simulink model "PC_MSFS_STATION"  (R2021b)
settings: Solver=FixedStepAuto  StartTime=0.0  StopTime=2000  FixedStep=0.03  RelTol=1e-3
undefined symbols (not defined in the file): CONTROL, DiscIntNeverNeededParam, f, MODEL, MODEL_INI
libraries: instrumentlib x42, SimConnectToolbox x6, simulink x4
(part 1 of 3)
settings Model: Creator=Andreas  LastModifiedBy=ae-dagbeyibor3
settings SolverCC: AlgebraicLoopSolver=TrustRegion
settings DebuggingCC: InheritedTsInSrcMsg=none  SFMachineParentedDataDiag=warning

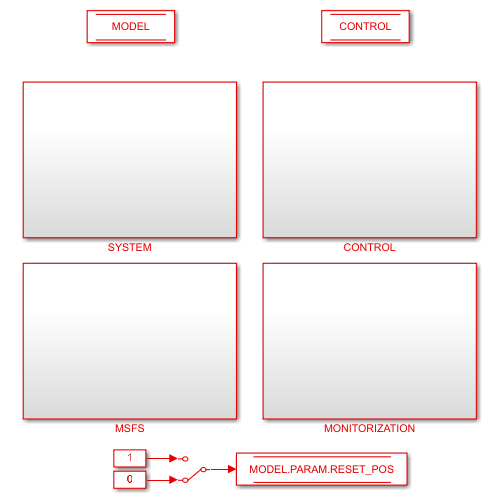
[thumbnail: Simulink's stored preview of the top-level diagram]
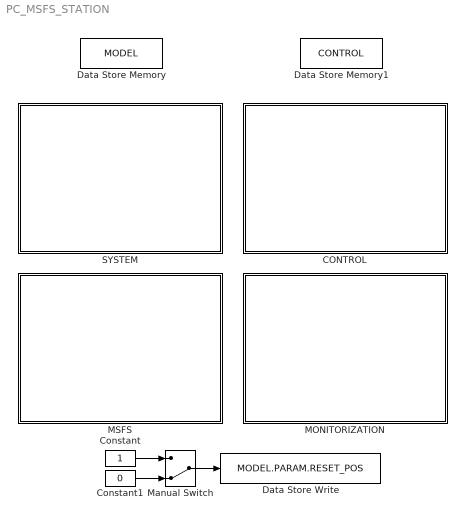
== system PC_MSFS_STATION ==
  CONTROL : Subsystem
  Constant : Constant  SampleTime=-1
  Constant1 : Constant  Value=0  SampleTime=-1
  Data Store Memory : DataStoreMemory  DataStoreName=MODEL  ReadBeforeWriteMsg=warning  WriteAfterWriteMsg=warning  WriteAfterReadMsg=warning  InitialValue=MODEL_INI  ShowAdditionalParam=off  OutDataTypeStr=Bus: MODEL_Bus
  Data Store Memory1 : DataStoreMemory  DataStoreName=CONTROL  ReadBeforeWriteMsg=warning  WriteAfterWriteMsg=warning  WriteAfterReadMsg=warning  InitialValue=CONTROL_INI  ShowAdditionalParam=off  OutDataTypeStr=Bus: CONTROL_Bus
  Data Store Write : DataStoreWrite  DataStoreName=MODEL  DataStoreElements=MODEL.PARAM.RESET_POS  IndexOptions=Index vector (dialog)  Indices=1  OutputSizes=1
  MONITORIZATION : Subsystem
  MSFS : Subsystem
  Manual Switch : ManualSwitch  CurrentSetting=0
  SYSTEM : Subsystem
  wires:
  Constant/1 -> Manual Switch/1
  Constant1/1 -> Manual Switch/2
  Manual Switch/1 -> Data Store Write/1

== system PC_MSFS_STATION/CONTROL ==
  ISR : Subsystem
  MEDEVAC : Subsystem  Commented=on

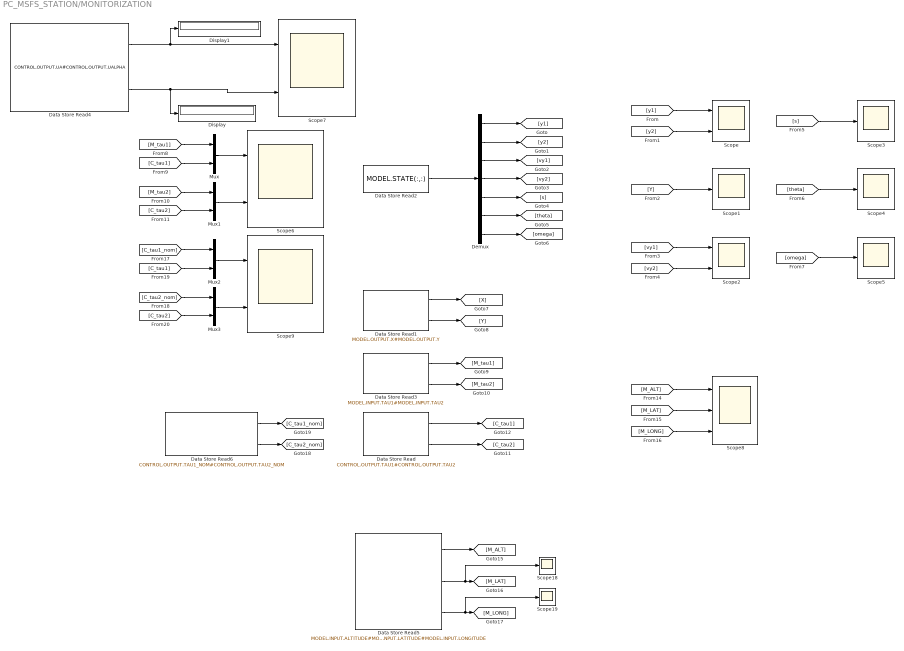
== system PC_MSFS_STATION/MONITORIZATION ==
  Data Store Read : DataStoreRead  DataStoreName=CONTROL  DataStoreElements=CONTROL.OUTPUT.TAU1#CONTROL.OUTPUT.TAU2  IndexOptions=Index vector (dialog)  Indices=1  OutputSizes=1
  Data Store Read1 : DataStoreRead  DataStoreName=MODEL  SampleTime=MODEL_INI.PARAM.SIM_SAMPLING_TIME  DataStoreElements=MODEL.OUTPUT.X#MODEL.OUTPUT.Y  IndexOptions=Index vector (dialog)  Indices=1  OutputSizes=1
  Data Store Read2 : DataStoreRead  DataStoreName=MODEL  SampleTime=MODEL_INI.PARAM.SIM_SAMPLING_TIME  DataStoreElements=MODEL.STATE(:,:)  IndexOptions=Index vector (dialog)  Indices=1  OutputSizes=1
  Data Store Read3 : DataStoreRead  DataStoreName=MODEL  SampleTime=MODEL_INI.PARAM.SIM_SAMPLING_TIME  DataStoreElements=MODEL.INPUT.TAU1#MODEL.INPUT.TAU2  IndexOptions=Index vector (dialog)  Indices=1  OutputSizes=1
  Data Store Read4 : DataStoreRead  DataStoreName=CONTROL  DataStoreElements=CONTROL.OUTPUT.UA#CONTROL.OUTPUT.UALPHA  IndexOptions=Index vector (dialog)  Indices=1  OutputSizes=1
  Data Store Read5 : DataStoreRead  DataStoreName=MODEL  SampleTime=MODEL_INI.PARAM.SIM_SAMPLING_TIME  DataStoreElements=MODEL.INPUT.ALTITUDE#MODEL.INPUT.LATITUDE#MODEL.INPUT.LONGITUDE  IndexOptions=Index vector (dialog)  Indices=1  OutputSizes=1
  Data Store Read6 : DataStoreRead  DataStoreName=CONTROL  DataStoreElements=CONTROL.OUTPUT.TAU1_NOM#CONTROL.OUTPUT.TAU2_NOM  IndexOptions=Index vector (dialog)  Indices=1  OutputSizes=1
  Demux : Demux  Outputs=7
  Display : Display
  Display1 : Display
  Mux{,1..3} (4 alike) : Mux  Inputs=2
  Scope{,2,6..7,9} (5 alike) : Scope  NumInputPorts=2
  Scope{1,3..5,18..19} (6 alike) : Scope
  Scope8 : Scope  NumInputPorts=3
  wires:
  Data Store Read2/1 -> Demux/1
  Demux/1 -> [y1]
  Demux/2 -> [y2]
  Demux/3 -> [vy1]
  Demux/4 -> [vy2]
  Demux/5 -> [s]
  Demux/6 -> [theta]
  Demux/7 -> [omega]
  [y1] -> Scope/1
  [y2] -> Scope/2
  Data Store Read1/1 -> [X]
  Data Store Read1/2 -> [Y]
  [Y] -> Scope1/1
  [vy2] -> Scope2/2
  [vy1] -> Scope2/1
  [s] -> Scope3/1
  [theta] -> Scope4/1
  [omega] -> Scope5/1
  Data Store Read3/1 -> [M_tau1]
  Data Store Read3/2 -> [M_tau2]
  Data Store Read/1 -> [C_tau1]
  Data Store Read/2 -> [C_tau2]
  Mux/1 -> Scope6/1
  Mux1/1 -> Scope6/2
  [M_tau1] -> Mux/1
  [M_tau2] -> Mux1/1
  [C_tau2] -> Mux1/2
  [C_tau1] -> Mux/2
  Data Store Read5/2 -> Scope18/1, [M_LAT]
  Data Store Read5/1 -> [M_ALT]
  Data Store Read5/3 -> Scope19/1, [M_LONG]
  [M_LAT] -> Scope8/2
  [M_ALT] -> Scope8/1
  [M_LONG] -> Scope8/3
  Data Store Read6/2 -> [C_tau2_nom]
  Data Store Read6/1 -> [C_tau1_nom]
  [C_tau1] -> Mux2/2
  [C_tau2] -> Mux3/2
  [C_tau2_nom] -> Mux3/1
  [C_tau1_nom] -> Mux2/1
  Mux3/1 -> Scope9/2
  Mux2/1 -> Scope9/1
  Data Store Read4/1 -> Display1/1, Scope7/1
  Data Store Read4/2 -> Display/1, Scope7/2

== system PC_MSFS_STATION/MSFS ==
  ISR : Subsystem
  MEDEVAC : Subsystem  Commented=on

== system PC_MSFS_STATION/SYSTEM ==
  ISR : Subsystem
  MEDEVAC : Subsystem  Commented=on

== system PC_MSFS_STATION/CONTROL/ISR ==
  Bus Selector : BusSelector  OutputSignals=STATE,INPUT.ALTITUDE
  Bus Selector1 : BusSelector  OutputSignals=PARAM.ALTITUDE
  CONTROL UPDATE : MATLAB Function  TreatAsAtomicUnit=on
  Data Store Read : DataStoreRead  DataStoreName=CONTROL  SampleTime=MODEL_INI.PARAM.SIM_SAMPLING_TIME  IndexOptions=Index vector (dialog)  Indices=1  OutputSizes=1
  Data Store Read1 : DataStoreRead  DataStoreName=MODEL  SampleTime=MODEL_INI.PARAM.SIM_SAMPLING_TIME  IndexOptions=Index vector (dialog)  Indices=1  OutputSizes=1
  Data Store Write : DataStoreWrite  DataStoreName=CONTROL  IndexOptions=Index vector (dialog)  Indices=1  OutputSizes=1
  Display : Display
  Scope : Scope
  Scope1 : Scope
  wires:
  Data Store Read1/1 -> Bus Selector/1
  Bus Selector1/1 -> Display/1, Scope1/1  "<ALTITUDE>"
  Data Store Read/1 -> CONTROL UPDATE/1(CONTROL_IN)
  CONTROL UPDATE/1(CONTROL) -> Bus Selector1/1, Data Store Write/1
  Bus Selector/1 -> CONTROL UPDATE/2(STATE)  "<STATE>"
  Bus Selector/2 -> CONTROL UPDATE/3(ALTITUDE_IN), Scope/1  "<ALTITUDE>"

== system PC_MSFS_STATION/CONTROL/MEDEVAC ==
  Bus Selector : BusSelector  OutputSignals=STATE,INPUT.ALTITUDE
  Bus Selector1 : BusSelector  OutputSignals=PARAM.ALTITUDE
  CONTROL UPDATE : MATLAB Function  TreatAsAtomicUnit=on
  Data Store Read : DataStoreRead  DataStoreName=CONTROL  SampleTime=MODEL_INI.PARAM.SIM_SAMPLING_TIME  IndexOptions=Index vector (dialog)  Indices=1  OutputSizes=1
  Data Store Read1 : DataStoreRead  DataStoreName=MODEL  SampleTime=MODEL_INI.PARAM.SIM_SAMPLING_TIME  IndexOptions=Index vector (dialog)  Indices=1  OutputSizes=1
  Data Store Write : DataStoreWrite  DataStoreName=CONTROL  IndexOptions=Index vector (dialog)  Indices=1  OutputSizes=1
  Display : Display
  Scope : Scope
  Scope1 : Scope
  wires:
  Bus Selector/2 -> Scope/1, CONTROL UPDATE/3(ALTITUDE_IN)  "<ALTITUDE>"
  Bus Selector/1 -> CONTROL UPDATE/2(STATE)  "<STATE>"
  CONTROL UPDATE/1(CONTROL) -> Data Store Write/1, Bus Selector1/1
  Data Store Read/1 -> CONTROL UPDATE/1(CONTROL_IN)
  Bus Selector1/1 -> Scope1/1, Display/1  "<ALTITUDE>"
  Data Store Read1/1 -> Bus Selector/1

== system PC_MSFS_STATION/MSFS/ISR ==
  COMMUNICATIONS : Subsystem
  Compare To Constant1 : simulink/Logic and Bit Operations/Compare To Constant  relop=>  const=0  OutDataTypeStr=boolean
  Compare To Constant4 : simulink/Logic and Bit Operations/Compare To Constant  relop===  const=0  OutDataTypeStr=boolean
  Data Store Read1 : DataStoreRead  DataStoreName=CONTROL  DataStoreElements=CONTROL.PARAM.FLIGHT_STATUS  IndexOptions=Index vector (dialog)  Indices=1  OutputSizes=1
  Data Store Read4 : DataStoreRead  DataStoreName=CONTROL  DataStoreElements=CONTROL.PARAM.FLIGHT_STATUS  IndexOptions=Index vector (dialog)  Indices=1  OutputSizes=1
  IN FLIGHT : Subsystem
  TAKE OFF TRIM : Subsystem
  wires:
  Data Store Read4/1 -> Compare To Constant4/1
  Compare To Constant1/1 -> IN FLIGHT/Enable
  Compare To Constant4/1 -> TAKE OFF TRIM/Enable
  Data Store Read1/1 -> Compare To Constant1/1

== system PC_MSFS_STATION/MSFS/MEDEVAC ==
  COMMUNICATIONS : Subsystem
  Compare To Constant1 : simulink/Logic and Bit Operations/Compare To Constant  relop=>  const=0  OutDataTypeStr=boolean
  Compare To Constant4 : simulink/Logic and Bit Operations/Compare To Constant  relop===  const=0  OutDataTypeStr=boolean
  Data Store Read1 : DataStoreRead  DataStoreName=CONTROL  DataStoreElements=CONTROL.PARAM.FLIGHT_STATUS  IndexOptions=Index vector (dialog)  Indices=1  OutputSizes=1
  Data Store Read4 : DataStoreRead  DataStoreName=CONTROL  DataStoreElements=CONTROL.PARAM.FLIGHT_STATUS  IndexOptions=Index vector (dialog)  Indices=1  OutputSizes=1
  IN FLIGHT : Subsystem
  TAKE OFF TRIM : Subsystem
  wires:
  Data Store Read1/1 -> Compare To Constant1/1
  Compare To Constant4/1 -> TAKE OFF TRIM/Enable
  Compare To Constant1/1 -> IN FLIGHT/Enable
  Data Store Read4/1 -> Compare To Constant4/1

== system PC_MSFS_STATION/SYSTEM/ISR ==
  Bus Selector2 : BusSelector  OutputSignals=OUTPUT.TAU1,OUTPUT.TAU2
  Bus Selector3 : BusSelector  OutputSignals=PARAM.FLIGHT_STATUS
  Data Store Read2 : DataStoreRead  DataStoreName=MODEL  SampleTime=MODEL_INI.PARAM.SIM_SAMPLING_TIME  IndexOptions=Index vector (dialog)  Indices=1  OutputSizes=1
  Data Store Read3 : DataStoreRead  DataStoreName=CONTROL  IndexOptions=Index vector (dialog)  Indices=1  OutputSizes=1
  Data Store Read4 : DataStoreRead  DataStoreName=CONTROL  DataStoreElements=CONTROL.PARAM.ALTITUDE  IndexOptions=Index vector (dialog)  Indices=1  OutputSizes=1
  Data Store Read5 : DataStoreRead  DataStoreName=CONTROL  IndexOptions=Index vector (dialog)  Indices=1  OutputSizes=1
  Data Store Read6 : DataStoreRead  DataStoreName=MODEL  DataStoreElements=MODEL.PARAM.RESET_POS  IndexOptions=Index vector (dialog)  Indices=1  OutputSizes=1
  Data Store Read8 : DataStoreRead  DataStoreName=MODEL  DataStoreElements=MODEL.PARAM.INIT_STATE(:,:)  IndexOptions=Index vector (dialog)  Indices=1  OutputSizes=1
  Data Store Write : DataStoreWrite  DataStoreName=MODEL  IndexOptions=Index vector (dialog)  Indices=1  OutputSizes=1
  Data Store Write2 : DataStoreWrite  DataStoreName=MODEL  DataStoreElements=MODEL.INPUT.TAU1#MODEL.INPUT.TAU2  IndexOptions=Index vector (dialog)  Indices=1  OutputSizes=1
  Data Store Write3 : DataStoreWrite  DataStoreName=MODEL  DataStoreElements=MODEL.PARAM.FLIGHT_STATUS  IndexOptions=Index vector (dialog)  Indices=1  OutputSizes=1
  Data Store Write4 : DataStoreWrite  DataStoreName=MODEL  DataStoreElements=MODEL.OUTPUT.ALTITUDE  IndexOptions=Index vector (dialog)  Indices=1  OutputSizes=1
  Demux : Demux  Outputs=7
  Discrete-Time Integrator : DiscreteIntegrator  ExternalReset=rising  InitialConditionSource=external  SampleTime=-1  ICPrevOutput=DiscIntNeverNeededParam  ICPrevScaledInput=DiscIntNeverNeededParam
  Display{,1,10..11,16..20} (9 alike) : Display
  Scope{,1..5,10..14} (11 alike) : Scope
  UNICYCLE MODEL : MATLAB Function  TreatAsAtomicUnit=on
  wires:
  Discrete-Time Integrator/1 -> Demux/1, UNICYCLE MODEL/1(STATE)
  UNICYCLE MODEL/2(MODEL) -> Data Store Write/1
  Data Store Read8/1 -> Discrete-Time Integrator/3
  UNICYCLE MODEL/1(STATE_DERIVATIVE) -> Discrete-Time Integrator/1
  Bus Selector2/2 -> Scope2/1, Data Store Write2/2  "<TAU2>"
  Demux/3 -> Scope10/1, Display16/1
  Bus Selector3/1 -> Display1/1, Data Store Write3/1, Scope1/1  "<FLIGHT_STATUS>"
  Bus Selector2/1 -> Scope3/1, Data Store Write2/1  "<TAU1>"
  Data Store Read4/1 -> Display/1, Scope/1, Data Store Write4/1
  Data Store Read3/1 -> Bus Selector3/1
  Demux/6 -> Scope13/1, Display19/1
  Demux/5 -> Scope12/1, Display18/1
  Data Store Read5/1 -> Bus Selector2/1
  Demux/1 -> Scope4/1, Display10/1
  Demux/7 -> Scope14/1, Display20/1
  Demux/2 -> Scope5/1, Display11/1
  Data Store Read2/1 -> UNICYCLE MODEL/2(MODEL_IN)
  Demux/4 -> Scope11/1, Display17/1
  Data Store Read6/1 -> Discrete-Time Integrator/2

== system PC_MSFS_STATION/SYSTEM/MEDEVAC ==
  Bus Selector2 : BusSelector  OutputSignals=OUTPUT.TAU1,OUTPUT.TAU2
  Bus Selector3 : BusSelector  OutputSignals=PARAM.FLIGHT_STATUS
  Data Store Read2 : DataStoreRead  DataStoreName=MODEL  SampleTime=MODEL_INI.PARAM.SIM_SAMPLING_TIME  IndexOptions=Index vector (dialog)  Indices=1  OutputSizes=1
  Data Store Read3 : DataStoreRead  DataStoreName=CONTROL  IndexOptions=Index vector (dialog)  Indices=1  OutputSizes=1
  Data Store Read4 : DataStoreRead  DataStoreName=CONTROL  DataStoreElements=CONTROL.PARAM.ALTITUDE  IndexOptions=Index vector (dialog)  Indices=1  OutputSizes=1
  Data Store Read5 : DataStoreRead  DataStoreName=CONTROL  IndexOptions=Index vector (dialog)  Indices=1  OutputSizes=1
  Data Store Read6 : DataStoreRead  DataStoreName=MODEL  DataStoreElements=MODEL.PARAM.RESET_POS  IndexOptions=Index vector (dialog)  Indices=1  OutputSizes=1
  Data Store Read8 : DataStoreRead  DataStoreName=MODEL  DataStoreElements=MODEL.PARAM.INIT_STATE(:,:)  IndexOptions=Index vector (dialog)  Indices=1  OutputSizes=1
  Data Store Write : DataStoreWrite  DataStoreName=MODEL  IndexOptions=Index vector (dialog)  Indices=1  OutputSizes=1
  Data Store Write2 : DataStoreWrite  DataStoreName=MODEL  DataStoreElements=MODEL.INPUT.TAU1#MODEL.INPUT.TAU2  IndexOptions=Index vector (dialog)  Indices=1  OutputSizes=1
  Data Store Write3 : DataStoreWrite  DataStoreName=MODEL  DataStoreElements=MODEL.PARAM.FLIGHT_STATUS  IndexOptions=Index vector (dialog)  Indices=1  OutputSizes=1
  Data Store Write4 : DataStoreWrite  DataStoreName=MODEL  DataStoreElements=MODEL.OUTPUT.ALTITUDE  IndexOptions=Index vector (dialog)  Indices=1  OutputSizes=1
  Demux : Demux  Outputs=7
  Discrete-Time Integrator : DiscreteIntegrator  ExternalReset=rising  InitialConditionSource=external  SampleTime=-1  ICPrevOutput=DiscIntNeverNeededParam  ICPrevScaledInput=DiscIntNeverNeededParam
  Display{,1,10..11,16..20} (9 alike) : Display
  Scope{,1..5,10..14} (11 alike) : Scope
  UNICYCLE MODEL : MATLAB Function  TreatAsAtomicUnit=on
  wires:
  Data Store Read6/1 -> Discrete-Time Integrator/2
  Demux/4 -> Display17/1, Scope11/1
  Data Store Read2/1 -> UNICYCLE MODEL/2(MODEL_IN)
  Demux/2 -> Display11/1, Scope5/1
  Demux/7 -> Display20/1, Scope14/1
  Demux/1 -> Display10/1, Scope4/1
  Data Store Read5/1 -> Bus Selector2/1
  Demux/5 -> Display18/1, Scope12/1
  Demux/6 -> Display19/1, Scope13/1
  Data Store Read3/1 -> Bus Selector3/1
  Data Store Read4/1 -> Data Store Write4/1, Scope/1, Display/1
  Bus Selector2/1 -> Data Store Write2/1, Scope3/1  "<TAU1>"
  Bus Selector3/1 -> Scope1/1, Data Store Write3/1, Display1/1  "<FLIGHT_STATUS>"
  Demux/3 -> Display16/1, Scope10/1
  Bus Selector2/2 -> Data Store Write2/2, Scope2/1  "<TAU2>"
  UNICYCLE MODEL/1(STATE_DERIVATIVE) -> Discrete-Time Integrator/1
  Data Store Read8/1 -> Discrete-Time Integrator/3
  UNICYCLE MODEL/2(MODEL) -> Data Store Write/1
  Discrete-Time Integrator/1 -> UNICYCLE MODEL/1(STATE), Demux/1

== system PC_MSFS_STATION/MSFS/ISR/COMMUNICATIONS ==
  LOCAL COMMUNICATIONS : Subsystem  Commented=on
  SERVER COMMUNICATIONS : Subsystem

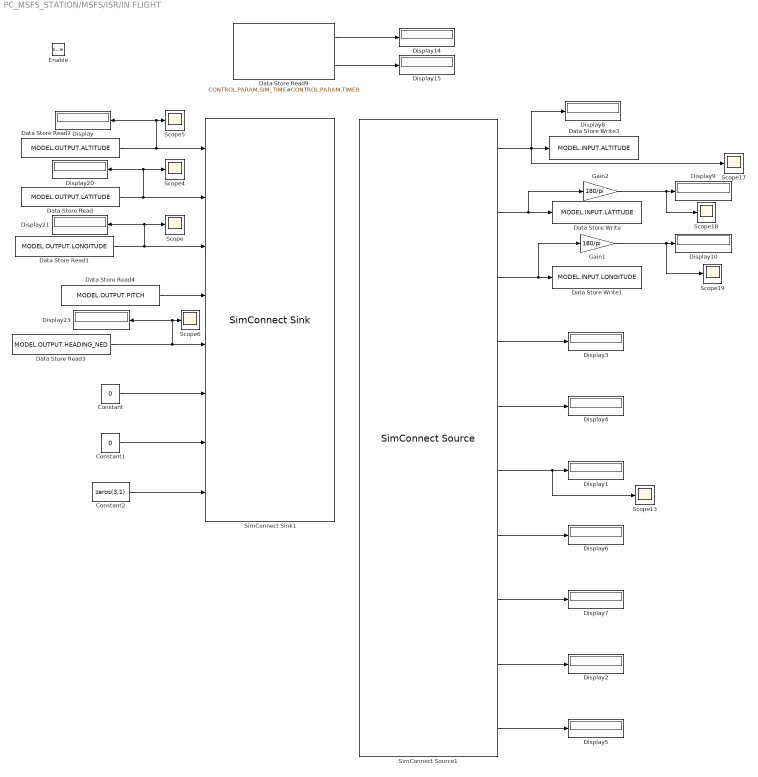
== system PC_MSFS_STATION/MSFS/ISR/IN FLIGHT ==
  Enable : EnablePort
  Constant : Constant  Value=0  SampleTime=-1
  Constant1 : Constant  Value=0  SampleTime=-1
  Constant2 : Constant  Value=zeros(3,1)  SampleTime=-1
  Data Store Read : DataStoreRead  DataStoreName=MODEL  DataStoreElements=MODEL.OUTPUT.LATITUDE  IndexOptions=Index vector (dialog)  Indices=1  OutputSizes=1
  Data Store Read1 : DataStoreRead  DataStoreName=MODEL  DataStoreElements=MODEL.OUTPUT.LONGITUDE  IndexOptions=Index vector (dialog)  Indices=1  OutputSizes=1
  Data Store Read2 : DataStoreRead  DataStoreName=MODEL  DataStoreElements=MODEL.OUTPUT.ALTITUDE  IndexOptions=Index vector (dialog)  Indices=1  OutputSizes=1
  Data Store Read3 : DataStoreRead  DataStoreName=MODEL  DataStoreElements=MODEL.OUTPUT.HEADING_NED  IndexOptions=Index vector (dialog)  Indices=1  OutputSizes=1
  Data Store Read4 : DataStoreRead  DataStoreName=MODEL  DataStoreElements=MODEL.OUTPUT.PITCH  IndexOptions=Index vector (dialog)  Indices=1  OutputSizes=1
  Data Store Read9 : DataStoreRead  DataStoreName=CONTROL  DataStoreElements=CONTROL.PARAM.SIM_TIME#CONTROL.PARAM.TIMER  IndexOptions=Index vector (dialog)  Indices=1  OutputSizes=1
  Data Store Write : DataStoreWrite  DataStoreName=MODEL  DataStoreElements=MODEL.INPUT.LATITUDE  IndexOptions=Index vector (dialog)  Indices=1  OutputSizes=1
  Data Store Write1 : DataStoreWrite  DataStoreName=MODEL  DataStoreElements=MODEL.INPUT.LONGITUDE  IndexOptions=Index vector (dialog)  Indices=1  OutputSizes=1
  Data Store Write3 : DataStoreWrite  DataStoreName=MODEL  DataStoreElements=MODEL.INPUT.ALTITUDE  IndexOptions=Index vector (dialog)  Indices=1  OutputSizes=1
  Display{,1..10,14..15,20..21,23} (16 alike) : Display
  Gain1 : Gain  Gain=180/pi
  Gain2 : Gain  Gain=180/pi
  Scope{,4..6,13,17..19} (8 alike) : Scope
  SimConnect Sink1 : SimConnectToolbox/SimConnect Sink  configurationIndex=0  connectionName=SimConnectSink  variables=|
      | PLANE ALTITUDE, FEET;
      | PLANE LATITUDE, RADIANS;
      | PLANE LONGITUDE, RADIANS;
      | PLANE PITCH DEGREES, RADIANS;
      | PLANE HEADING DEGREES TRUE, RADIANS;
      | PLANE BANK DEGREES, RADIANS;
      | AILERON POSITION, POSITION;
      | AILERON TRIM PCT, PERCENT;
      settings: SourceProductName=SimConnect Toolbox
      mask Display:
      | % This is a new mask on top of the base mask.
      | % Use "View base mask" link below to see the base mask.
      | %port_label('input', 1, 'Rudder Trim', 'texmode', 'on')
      | port_label('input', 1, 'PLANE ALTITUDE, FEET', 'texmode', 'on')
      | port_label('input', 2, 'PLANE LATITUDE, RADIANS', 'texmode', 'on')
      | port_label('input', 3, 'PLANE LONGITUDE, RADIANS', 'texmode', 'on')
      | port_label('input', 4, 'PITCH DEGREES, RADIANS', 'texmode', 'on')
      | port_label('input', 5, 'HEADING DEGREES TRUE, RADIANS', 'texmode', 'on')
      | port_label('input', 6, 'PLANE BANK DEGREES, RADIANS;', 'texmode', 'on')
      | port_label('input', 7, 'AILERON POSITION, POSITION', 'texmode', 'on')
      | port_label('input', 8, 'AILERON TRIM PCT, PERCENT OVER 100', 'texmode', 'on')
  SimConnect Source1 : SimConnectToolbox/SimConnect Source  configurationIndex=0  connectionName=SimConnectSource  variables=|
      | PLANE ALTITUDE, FEET;
      | PLANE LATITUDE, RADIANS;
      | PLANE LONGITUDE, RADIANS;
      | ROTATION VELOCITY BODY X, FEET PER SECOND;
      | PLANE PITCH DEGREES, RADIANS;
      | PLANE HEADING DEGREES TRUE, RADIANS;
      | PLANE HEADING DEGREES MAGNETIC, RADIANS;
      | PLANE HEADING DEGREES GYRO, DEGREES;
      | AILERON POSITION, POSITION;
      | AILERON TRIM PCT, PERCENT OVER 100;
      settings: SourceProductName=SimConnect Toolbox
      mask Display:
      | % This is a new mask on top of the base mask.
      | % Use "View base mask" link below to see the base mask.
      | % port_label('output', 1, 'g', 'texmode', 'on')
      | port_label('output', 1, 'PLANE ALTITUDE, FEET', 'texmode', 'on')
      | port_label('output', 2, 'PLANE LATITUDE, RADIANS', 'texmode', 'on')
      | port_label('output', 3, 'PLANE LONGITUDE, RADIANS', 'texmode', 'on')
      | port_label('output', 4, 'VELOCITY BODY X, FEET PER SECOND', 'texmode', 'on')
      | port_label('output', 5, 'PITCH DEGREES, RADIANS', 'texmode', 'on')
      | port_label('output', 6, 'HEADING DEGREES TRUE, RADIANS', 'texmode', 'on')
      | port_label('output', 7, 'HEADING DEGREES MAGNETIC, RADIANS', 'texmode', 'on')
      | port_label('output', 8, 'HEADING DEGREES GYRO, DEGREES', 'texmode', 'on')
      | port_label('output', 9, 'AILERON POSITION, POSITION', 'texmode', 'on')
      | port_label('output', 10, 'AILERON TRIM PCT, PERCENT OVER 100', 'texmode', 'on')
  wires:
  Constant2/1 -> SimConnect Sink1/8
  SimConnect Source1/9 -> Display2/1
  Constant/1 -> SimConnect Sink1/6
  Data Store Read1/1 -> Display21/1, Scope/1, SimConnect Sink1/3
  Constant1/1 -> SimConnect Sink1/7
  SimConnect Source1/5 -> Display4/1
  SimConnect Source1/8 -> Display7/1
  SimConnect Source1/6 -> Scope13/1, Display1/1
  Data Store Read2/1 -> Display/1, Scope5/1, SimConnect Sink1/1
  Data Store Read/1 -> Display20/1, Scope4/1, SimConnect Sink1/2
  Data Store Read4/1 -> SimConnect Sink1/4
  SimConnect Source1/4 -> Display3/1
  SimConnect Source1/1 -> Data Store Write3/1, Display8/1, Scope17/1
  SimConnect Source1/7 -> Display6/1
  SimConnect Source1/10 -> Display5/1
  Data Store Read9/1 -> Display14/1
  Data Store Read9/2 -> Display15/1
  Data Store Read3/1 -> Display23/1, Scope6/1, SimConnect Sink1/5
  SimConnect Source1/2 -> Gain2/1, Data Store Write/1
  SimConnect Source1/3 -> Data Store Write1/1, Gain1/1
  Gain2/1 -> Scope18/1, Display9/1
  Gain1/1 -> Scope19/1, Display10/1

== system PC_MSFS_STATION/MSFS/ISR/TAKE OFF TRIM ==
  Enable : EnablePort
  Data Store Write : DataStoreWrite  DataStoreName=MODEL  DataStoreElements=MODEL.INPUT.LATITUDE  IndexOptions=Index vector (dialog)  Indices=1  OutputSizes=1
  Data Store Write1 : DataStoreWrite  DataStoreName=MODEL  DataStoreElements=MODEL.INPUT.LONGITUDE  IndexOptions=Index vector (dialog)  Indices=1  OutputSizes=1
  Data Store Write2 : DataStoreWrite  DataStoreName=MODEL  DataStoreElements=MODEL.INPUT.ALTITUDE  IndexOptions=Index vector (dialog)  Indices=1  OutputSizes=1
  Display1 : Display
  Display2 : Display
  Display3 : Display
  SimConnect Source1 : SimConnectToolbox/SimConnect Source  configurationIndex=0  connectionName=SimConnectSource  variables=|
      | PLANE ALTITUDE, FEET;
      | PLANE LATITUDE, RADIANS;
      | PLANE LONGITUDE, RADIANS;
      settings: SourceProductName=SimConnect Toolbox
      mask Display:
      | % This is a new mask on top of the base mask.
      | % Use "View base mask" link below to see the base mask.
      | % port_label('output', 1, 'g', 'texmode', 'on')
      | port_label('output', 1, 'PLANE ALTITUDE, FEET', 'texmode', 'on')
      | port_label('output', 2, 'PLANE LATITUDE, RADIANS', 'texmode', 'on')
      | port_label('output', 3, 'PLANE LONGITUDE, RADIANS', 'texmode', 'on')
  wires:
  SimConnect Source1/2 -> Data Store Write/1, Display2/1
  SimConnect Source1/1 -> Display3/1, Data Store Write2/1
  SimConnect Source1/3 -> Display1/1, Data Store Write1/1

== system PC_MSFS_STATION/MSFS/MEDEVAC/COMMUNICATIONS ==
  LOCAL COMMUNICATIONS : Subsystem  Commented=on
  SERVER COMMUNICATIONS : Subsystem

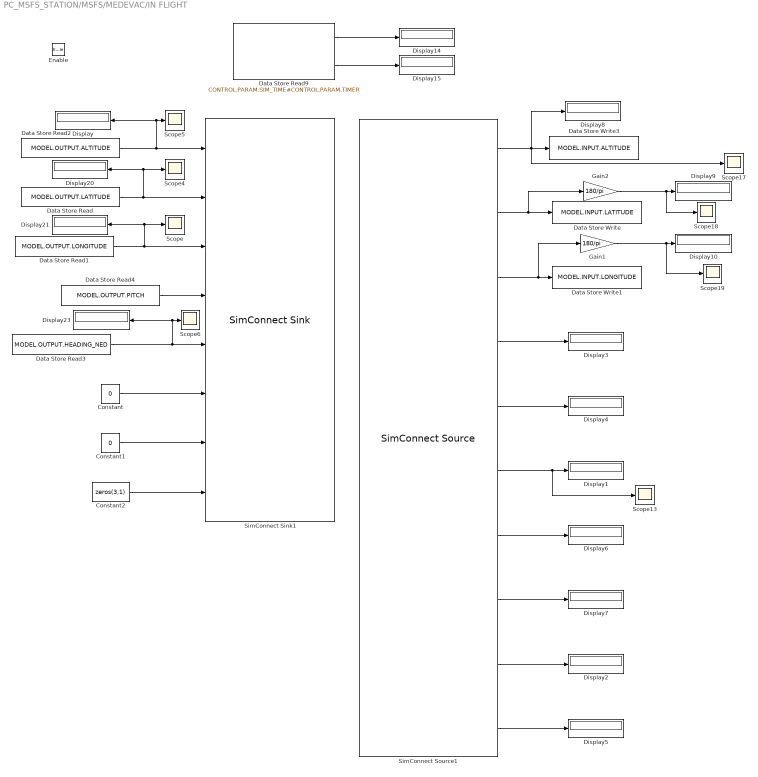
== system PC_MSFS_STATION/MSFS/MEDEVAC/IN FLIGHT ==
  Enable : EnablePort
  Constant : Constant  Value=0  SampleTime=-1
  Constant1 : Constant  Value=0  SampleTime=-1
  Constant2 : Constant  Value=zeros(3,1)  SampleTime=-1
  Data Store Read : DataStoreRead  DataStoreName=MODEL  DataStoreElements=MODEL.OUTPUT.LATITUDE  IndexOptions=Index vector (dialog)  Indices=1  OutputSizes=1
  Data Store Read1 : DataStoreRead  DataStoreName=MODEL  DataStoreElements=MODEL.OUTPUT.LONGITUDE  IndexOptions=Index vector (dialog)  Indices=1  OutputSizes=1
  Data Store Read2 : DataStoreRead  DataStoreName=MODEL  DataStoreElements=MODEL.OUTPUT.ALTITUDE  IndexOptions=Index vector (dialog)  Indices=1  OutputSizes=1
  Data Store Read3 : DataStoreRead  DataStoreName=MODEL  DataStoreElements=MODEL.OUTPUT.HEADING_NED  IndexOptions=Index vector (dialog)  Indices=1  OutputSizes=1
  Data Store Read4 : DataStoreRead  DataStoreName=MODEL  DataStoreElements=MODEL.OUTPUT.PITCH  IndexOptions=Index vector (dialog)  Indices=1  OutputSizes=1
  Data Store Read9 : DataStoreRead  DataStoreName=CONTROL  DataStoreElements=CONTROL.PARAM.SIM_TIME#CONTROL.PARAM.TIMER  IndexOptions=Index vector (dialog)  Indices=1  OutputSizes=1
  Data Store Write : DataStoreWrite  DataStoreName=MODEL  DataStoreElements=MODEL.INPUT.LATITUDE  IndexOptions=Index vector (dialog)  Indices=1  OutputSizes=1
  Data Store Write1 : DataStoreWrite  DataStoreName=MODEL  DataStoreElements=MODEL.INPUT.LONGITUDE  IndexOptions=Index vector (dialog)  Indices=1  OutputSizes=1
  Data Store Write3 : DataStoreWrite  DataStoreName=MODEL  DataStoreElements=MODEL.INPUT.ALTITUDE  IndexOptions=Index vector (dialog)  Indices=1  OutputSizes=1
  Display{,1..10,14..15,20..21,23} (16 alike) : Display
  Gain1 : Gain  Gain=180/pi
  Gain2 : Gain  Gain=180/pi
  Scope{,4..6,13,17..19} (8 alike) : Scope
  SimConnect Sink1 : SimConnectToolbox/SimConnect Sink  configurationIndex=0  connectionName=SimConnectSink  variables=|
      | PLANE ALTITUDE, FEET;
      | PLANE LATITUDE, RADIANS;
      | PLANE LONGITUDE, RADIANS;
      | PLANE PITCH DEGREES, RADIANS;
      | PLANE HEADING DEGREES TRUE, RADIANS;
      | PLANE BANK DEGREES, RADIANS;
      | AILERON POSITION, POSITION;
      | AILERON TRIM PCT, PERCENT;
      settings: SourceProductName=SimConnect Toolbox
      mask Display:
      | % This is a new mask on top of the base mask.
      | % Use "View base mask" link below to see the base mask.
      | %port_label('input', 1, 'Rudder Trim', 'texmode', 'on')
      | port_label('input', 1, 'PLANE ALTITUDE, FEET', 'texmode', 'on')
      | port_label('input', 2, 'PLANE LATITUDE, RADIANS', 'texmode', 'on')
      | port_label('input', 3, 'PLANE LONGITUDE, RADIANS', 'texmode', 'on')
      | port_label('input', 4, 'PITCH DEGREES, RADIANS', 'texmode', 'on')
      | port_label('input', 5, 'HEADING DEGREES TRUE, RADIANS', 'texmode', 'on')
      | port_label('input', 6, 'PLANE BANK DEGREES, RADIANS;', 'texmode', 'on')
      | port_label('input', 7, 'AILERON POSITION, POSITION', 'texmode', 'on')
      | port_label('input', 8, 'AILERON TRIM PCT, PERCENT OVER 100', 'texmode', 'on')
  SimConnect Source1 : SimConnectToolbox/SimConnect Source  configurationIndex=0  connectionName=SimConnectSource  variables=|
      | PLANE ALTITUDE, FEET;
      | PLANE LATITUDE, RADIANS;
      | PLANE LONGITUDE, RADIANS;
      | ROTATION VELOCITY BODY X, FEET PER SECOND;
      | PLANE PITCH DEGREES, RADIANS;
      | PLANE HEADING DEGREES TRUE, RADIANS;
      | PLANE HEADING DEGREES MAGNETIC, RADIANS;
      | PLANE HEADING DEGREES GYRO, DEGREES;
      | AILERON POSITION, POSITION;
      | AILERON TRIM PCT, PERCENT OVER 100;
      settings: SourceProductName=SimConnect Toolbox
      mask Display:
      | % This is a new mask on top of the base mask.
      | % Use "View base mask" link below to see the base mask.
      | % port_label('output', 1, 'g', 'texmode', 'on')
      | port_label('output', 1, 'PLANE ALTITUDE, FEET', 'texmode', 'on')
      | port_label('output', 2, 'PLANE LATITUDE, RADIANS', 'texmode', 'on')
      | port_label('output', 3, 'PLANE LONGITUDE, RADIANS', 'texmode', 'on')
      | port_label('output', 4, 'VELOCITY BODY X, FEET PER SECOND', 'texmode', 'on')
      | port_label('output', 5, 'PITCH DEGREES, RADIANS', 'texmode', 'on')
      | port_label('output', 6, 'HEADING DEGREES TRUE, RADIANS', 'texmode', 'on')
      | port_label('output', 7, 'HEADING DEGREES MAGNETIC, RADIANS', 'texmode', 'on')
      | port_label('output', 8, 'HEADING DEGREES GYRO, DEGREES', 'texmode', 'on')
      | port_label('output', 9, 'AILERON POSITION, POSITION', 'texmode', 'on')
      | port_label('output', 10, 'AILERON TRIM PCT, PERCENT OVER 100', 'texmode', 'on')
  wires:
  Gain1/1 -> Display10/1, Scope19/1
  Gain2/1 -> Display9/1, Scope18/1
  SimConnect Source1/3 -> Gain1/1, Data Store Write1/1
  SimConnect Source1/2 -> Data Store Write/1, Gain2/1
  Data Store Read3/1 -> SimConnect Sink1/5, Scope6/1, Display23/1
  Data Store Read9/2 -> Display15/1
  Data Store Read9/1 -> Display14/1
  SimConnect Source1/10 -> Display5/1
  SimConnect Source1/7 -> Display6/1
  SimConnect Source1/1 -> Scope17/1, Display8/1, Data Store Write3/1
  SimConnect Source1/4 -> Display3/1
  Data Store Read4/1 -> SimConnect Sink1/4
  Data Store Read/1 -> SimConnect Sink1/2, Scope4/1, Display20/1
  Data Store Read2/1 -> SimConnect Sink1/1, Scope5/1, Display/1
  SimConnect Source1/6 -> Display1/1, Scope13/1
  SimConnect Source1/8 -> Display7/1
  SimConnect Source1/5 -> Display4/1
  Constant1/1 -> SimConnect Sink1/7
  Data Store Read1/1 -> SimConnect Sink1/3, Scope/1, Display21/1
  Constant/1 -> SimConnect Sink1/6
  SimConnect Source1/9 -> Display2/1
  Constant2/1 -> SimConnect Sink1/8

== system PC_MSFS_STATION/MSFS/MEDEVAC/TAKE OFF TRIM ==
  Enable : EnablePort
  Data Store Write : DataStoreWrite  DataStoreName=MODEL  DataStoreElements=MODEL.INPUT.LATITUDE  IndexOptions=Index vector (dialog)  Indices=1  OutputSizes=1
  Data Store Write1 : DataStoreWrite  DataStoreName=MODEL  DataStoreElements=MODEL.INPUT.LONGITUDE  IndexOptions=Index vector (dialog)  Indices=1  OutputSizes=1
  Data Store Write2 : DataStoreWrite  DataStoreName=MODEL  DataStoreElements=MODEL.INPUT.ALTITUDE  IndexOptions=Index vector (dialog)  Indices=1  OutputSizes=1
  Display1 : Display
  Display2 : Display
  Display3 : Display
  SimConnect Source1 : SimConnectToolbox/SimConnect Source  configurationIndex=0  connectionName=SimConnectSource  variables=|
      | PLANE ALTITUDE, FEET;
      | PLANE LATITUDE, RADIANS;
      | PLANE LONGITUDE, RADIANS;
      settings: SourceProductName=SimConnect Toolbox
      mask Display:
      | % This is a new mask on top of the base mask.
      | % Use "View base mask" link below to see the base mask.
      | % port_label('output', 1, 'g', 'texmode', 'on')
      | port_label('output', 1, 'PLANE ALTITUDE, FEET', 'texmode', 'on')
      | port_label('output', 2, 'PLANE LATITUDE, RADIANS', 'texmode', 'on')
      | port_label('output', 3, 'PLANE LONGITUDE, RADIANS', 'texmode', 'on')
  wires:
  SimConnect Source1/3 -> Data Store Write1/1, Display1/1
  SimConnect Source1/1 -> Data Store Write2/1, Display3/1
  SimConnect Source1/2 -> Display2/1, Data Store Write/1

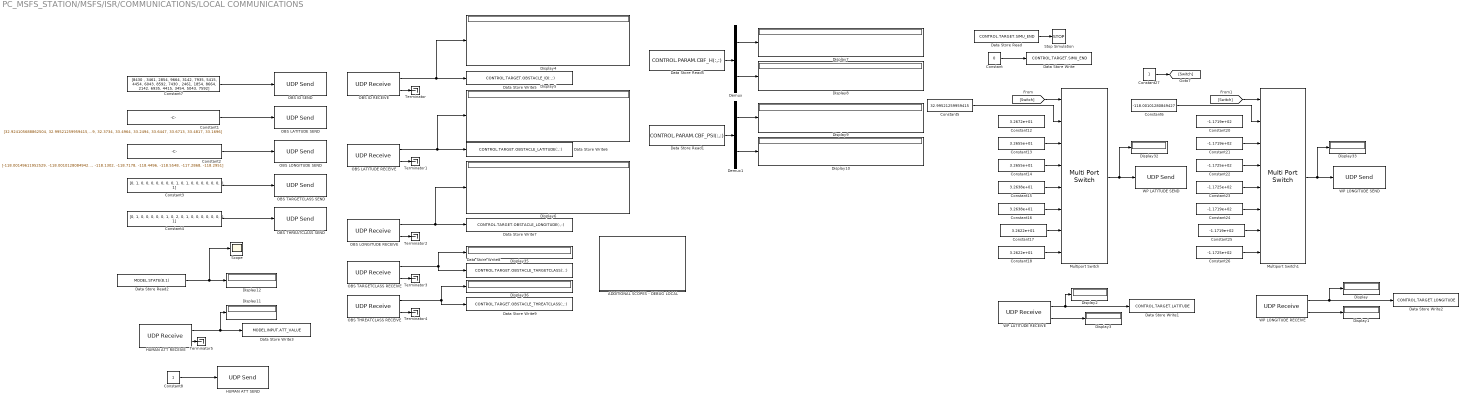
== system PC_MSFS_STATION/MSFS/ISR/COMMUNICATIONS/LOCAL COMMUNICATIONS ==
  ADDITIONAL SCOPES - DEBUG LOCAL : Subsystem
  Constant : Constant  Value=0  SampleTime=-1
  Constant1 : Constant  Value=[32.924105688862504, 32.99521259959415, 33.02158942564577, 32.91934321241453, 33.03164479405805, 33.006944746948776, 33.04647050546855, 33.04913481714204, 33.0301654991582, 32.99895800903812, 32.4211, 33.1321, 33.3959, 32.3734, 33.4964, 33.2494, 33.6447, 33.6713, 33.4817, 33.1696]  VectorParams1D=off  SampleTime=-1
  Constant12 : Constant  Value=3.2672e+01  SampleTime=0.03
  Constant13 : Constant  Value=3.2655e+01  SampleTime=0.03
  Constant14 : Constant  Value=3.2655e+01  SampleTime=0.03
  Constant15 : Constant  Value=3.2638e+01  SampleTime=0.03
  Constant16 : Constant  Value=3.2638e+01  SampleTime=0.03
  Constant17 : Constant  Value=3.2622e+01  SampleTime=0.03
  Constant18 : Constant  Value=3.2622e+01  SampleTime=0.03
  Constant2 : Constant  Value=[-118.00149611952529, -118.00101280849427, -117.96213226450607, -117.99775003148243, -117.9950188692361, -118.05377736883983, -118.02695832792669, -118.03747541511804, -117.91067889321968, -118.01150525972992, -118.1950, -118.1901, -117.8013, -118.1575, -118.1302, -118.7178, -118.4496, -118.5548, -117.2868, -118.2951]  SampleTime=-1
  Constant{20..21,24..25} (4 alike) : Constant  Value=-1.1719e+02  SampleTime=0.03
  Constant22 : Constant  Value=-1.1725e+02  SampleTime=0.03
  Constant23 : Constant  Value=-1.1725e+02  SampleTime=0.03
  Constant26 : Constant  Value=-1.1725e+02  SampleTime=0.03
  Constant27 : Constant  SampleTime=-1
  Constant3 : Constant  Value=[0, 1, 0, 0, 0, 0, 0, 0, 0, 1, 0, 1, 0, 0, 0, 0, 0, 0, 0, 1]  SampleTime=-1
  Constant4 : Constant  Value=[0, 1, 0, 0, 0, 0, 0, 1, 0, 2, 0, 1, 0, 0, 0, 0, 0, 0, 0, 1]  SampleTime=-1
  Constant5 : Constant  Value=32.99521259959415  SampleTime=0.03
  Constant6 : Constant  Value=-118.00101280849427  SampleTime=0.03
  Constant7 : Constant  Value=[8430 , 3461, 2854, 9664, 3142, 7935, 5415, 4454, 6043, 8592, 7430 , 2461, 1854, 8664, 2142, 6935, 4415, 3454, 5043, 7592]  SampleTime=-1
  Constant8 : Constant  SampleTime=-1
  Data Store Read : DataStoreRead  DataStoreName=CONTROL  DataStoreElements=CONTROL.TARGET.SIMU_END  IndexOptions=Index vector (dialog)  Indices=1  OutputSizes=1
  Data Store Read1 : DataStoreRead  DataStoreName=CONTROL  DataStoreElements=CONTROL.PARAM.CBF_PSI(:,:)  IndexOptions=Index vector (dialog)  Indices=1  OutputSizes=1
  Data Store Read2 : DataStoreRead  DataStoreName=MODEL  DataStoreElements=MODEL.STATE(8,1)  IndexOptions=Index vector (dialog)  Indices=1  OutputSizes=1
  Data Store Read5 : DataStoreRead  DataStoreName=CONTROL  DataStoreElements=CONTROL.PARAM.CBF_H(:,:)  IndexOptions=Index vector (dialog)  Indices=1  OutputSizes=1
  Data Store Write : DataStoreWrite  DataStoreName=CONTROL  DataStoreElements=CONTROL.TARGET.SIMU_END  IndexOptions=Index vector (dialog)  Indices=1  OutputSizes=1
  Data Store Write1 : DataStoreWrite  DataStoreName=CONTROL  DataStoreElements=CONTROL.TARGET.LATITUDE  IndexOptions=Index vector (dialog)  Indices=1  OutputSizes=1
  Data Store Write2 : DataStoreWrite  DataStoreName=CONTROL  DataStoreElements=CONTROL.TARGET.LONGITUDE  IndexOptions=Index vector (dialog)  Indices=1  OutputSizes=1
  Data Store Write3 : DataStoreWrite  DataStoreName=MODEL  DataStoreElements=MODEL.INPUT.ATT_VALUE  IndexOptions=Index vector (dialog)  Indices=1  OutputSizes=1
  Data Store Write5 : DataStoreWrite  DataStoreName=CONTROL  DataStoreElements=CONTROL.TARGET.OBSTACLE_ID(:,:)  IndexOptions=Index vector (dialog)  Indices=1  OutputSizes=1
  Data Store Write6 : DataStoreWrite  DataStoreName=CONTROL  DataStoreElements=CONTROL.TARGET.OBSTACLE_LATITUDE(:,:)  IndexOptions=Index vector (dialog)  Indices=1  OutputSizes=1
  Data Store Write7 : DataStoreWrite  DataStoreName=CONTROL  DataStoreElements=CONTROL.TARGET.OBSTACLE_LONGITUDE(:,:)  IndexOptions=Index vector (dialog)  Indices=1  OutputSizes=1
  Data Store Write8 : DataStoreWrite  DataStoreName=CONTROL  DataStoreElements=CONTROL.TARGET.OBSTACLE_TARGETCLASS(:,:)  IndexOptions=Index vector (dialog)  Indices=1  OutputSizes=1
  Data Store Write9 : DataStoreWrite  DataStoreName=CONTROL  DataStoreElements=CONTROL.TARGET.OBSTACLE_THREATCLASS(:,:)  IndexOptions=Index vector (dialog)  Indices=1  OutputSizes=1
  Demux : Demux  Outputs=2
  Demux1 : Demux  Outputs=2
  Display{,1..12,32..33,35..36} (17 alike) : Display
  HUMAN ATT RECEIVE : instrumentlib/UDP Receive  Host=127.0.0.1  Port=7083  LocalPort=7082  EnablePortSharing=off  GetLatestData=off  DataSize="[1  1]"  DataType=double  ASCIIFormatting=%f,  Terminator=LF  ByteOrder=BigEndian  EnableBlockingMode=off  Timeout=10  SampleTime=-1  LocalAddress=127.0.0.1
  HUMAN ATT SEND : instrumentlib/UDP Send  Host=127.0.0.1  Port=7082  LocalPort=7083  EnablePortSharing=off  ByteOrder=BigEndian  OutputDatagramPacketSize=512  EnableBlockingMode=on  LocalAddress=127.0.0.1
  Multiport Switch : MultiPortSwitch  Inputs=7
  Multiport Switch1 : MultiPortSwitch  Inputs=7
  OBS ID RECEIVE : instrumentlib/UDP Receive  Host=127.0.0.1  Port=8081  LocalPort=8082  EnablePortSharing=off  GetLatestData=off  DataSize="[20   1]"  DataType=double  ASCIIFormatting=%f,  Terminator=LF  ByteOrder=BigEndian  EnableBlockingMode=off  Timeout=10  SampleTime=-1  LocalAddress=127.0.0.1
  OBS ID SEND : instrumentlib/UDP Send  Host=127.0.0.1  Port=8082  LocalPort=8081  EnablePortSharing=off  ByteOrder=BigEndian  OutputDatagramPacketSize=512  EnableBlockingMode=on  LocalAddress=127.0.0.1
  OBS LATITUDE RECEIVE : instrumentlib/UDP Receive  Host=127.0.0.1  Port=8083  LocalPort=8084  EnablePortSharing=off  GetLatestData=off  DataSize="[20   1]"  DataType=double  ASCIIFormatting=%f,  Terminator=LF  ByteOrder=BigEndian  EnableBlockingMode=off  Timeout=10  SampleTime=-1  LocalAddress=127.0.0.1
  OBS LATITUDE SEND : instrumentlib/UDP Send  Host=127.0.0.1  Port=8084  LocalPort=8083  EnablePortSharing=off  ByteOrder=BigEndian  OutputDatagramPacketSize=512  EnableBlockingMode=on  LocalAddress=127.0.0.1
  OBS LONGITUDE RECEIVE : instrumentlib/UDP Receive  Host=127.0.0.1  Port=8085  LocalPort=8086  EnablePortSharing=off  GetLatestData=off  DataSize="[20   1]"  DataType=double  ASCIIFormatting=%f,  Terminator=LF  ByteOrder=BigEndian  EnableBlockingMode=off  Timeout=10  SampleTime=-1  LocalAddress=127.0.0.1
  OBS LONGITUDE SEND : instrumentlib/UDP Send  Host=127.0.0.1  Port=8086  LocalPort=8085  EnablePortSharing=off  ByteOrder=BigEndian  OutputDatagramPacketSize=512  EnableBlockingMode=on  LocalAddress=127.0.0.1
  OBS TARGETCLASS RECEIVE : instrumentlib/UDP Receive  Host=127.0.0.1  Port=7087  LocalPort=7088  EnablePortSharing=off  GetLatestData=off  DataSize="[20   1]"  DataType=double  ASCIIFormatting=%f,  Terminator=LF  ByteOrder=BigEndian  EnableBlockingMode=off  Timeout=10  SampleTime=-1  LocalAddress=127.0.0.1
  OBS TARGETCLASS SEND : instrumentlib/UDP Send  Host=127.0.0.1  Port=7088  LocalPort=7087  EnablePortSharing=off  ByteOrder=BigEndian  OutputDatagramPacketSize=512  EnableBlockingMode=on  LocalAddress=127.0.0.1
  OBS THREATCLASS RECEIVE : instrumentlib/UDP Receive  Host=127.0.0.1  Port=7089  LocalPort=7080  EnablePortSharing=off  GetLatestData=off  DataSize="[20   1]"  DataType=double  ASCIIFormatting=%f,  Terminator=LF  ByteOrder=BigEndian  EnableBlockingMode=off  Timeout=10  SampleTime=-1  LocalAddress=127.0.0.1
  OBS THREATCLASS SEND : instrumentlib/UDP Send  Host=127.0.0.1  Port=7080  LocalPort=7089  EnablePortSharing=off  ByteOrder=BigEndian  OutputDatagramPacketSize=512  EnableBlockingMode=on  LocalAddress=127.0.0.1
  Scope : Scope
  Stop Simulation : Stop
  Terminator{,1..5} (6 alike) : Terminator
  WP LATITUDE RECEIVE : instrumentlib/UDP Receive  Host=127.0.0.1  Port=8087  LocalPort=8080  EnablePortSharing=off  GetLatestData=off  DataSize=[1 1]  DataType=double  ASCIIFormatting=%f,  Terminator=LF  ByteOrder=BigEndian  EnableBlockingMode=off  Timeout=10  SampleTime=-1  LocalAddress=127.0.0.1
  WP LATITUDE SEND : instrumentlib/UDP Send  Host=127.0.0.1  Port=8080  LocalPort=8087  EnablePortSharing=off  ByteOrder=BigEndian  OutputDatagramPacketSize=512  EnableBlockingMode=on  LocalAddress=127.0.0.1
  WP LONGITUDE RECEIVE : instrumentlib/UDP Receive  Host=127.0.0.1  Port=8089  LocalPort=8088  EnablePortSharing=off  GetLatestData=off  DataSize=[1 1]  DataType=double  ASCIIFormatting=%f,  Terminator=LF  ByteOrder=BigEndian  EnableBlockingMode=off  Timeout=10  SampleTime=-1  LocalAddress=127.0.0.1
  WP LONGITUDE SEND : instrumentlib/UDP Send  Host=127.0.0.1  Port=8088  LocalPort=8089  EnablePortSharing=off  ByteOrder=BigEndian  OutputDatagramPacketSize=512  EnableBlockingMode=on  LocalAddress=127.0.0.1
  wires:
  WP LATITUDE RECEIVE/2 -> Display3/1
  WP LATITUDE RECEIVE/1 -> Display2/1, Data Store Write1/1
  WP LONGITUDE RECEIVE/1 -> Data Store Write2/1, Display/1
  WP LONGITUDE RECEIVE/2 -> Display1/1
  Data Store Read/1 -> Stop Simulation/1
  Constant/1 -> Data Store Write/1
  [Switch] -> Multiport Switch/1
  Constant13/1 -> Multiport Switch/3
  Constant14/1 -> Multiport Switch/4
  Constant15/1 -> Multiport Switch/5
  Constant16/1 -> Multiport Switch/6
  Constant17/1 -> Multiport Switch/7
  Constant18/1 -> Multiport Switch/8
  Multiport Switch/1 -> WP LATITUDE SEND/1, Display32/1
  Multiport Switch1/1 -> WP LONGITUDE SEND/1, Display33/1
  Constant26/1 -> Multiport Switch1/8
  Constant25/1 -> Multiport Switch1/7
  Constant24/1 -> Multiport Switch1/6
  Constant23/1 -> Multiport Switch1/5
  Constant22/1 -> Multiport Switch1/4
  Constant21/1 -> Multiport Switch1/3
  [Switch] -> Multiport Switch1/1
  Constant27/1 -> [Switch]
  OBS ID RECEIVE/1 -> Data Store Write5/1, Display4/1
  OBS LATITUDE RECEIVE/1 -> Display5/1, Data Store Write6/1
  OBS LONGITUDE RECEIVE/1 -> Display6/1, Data Store Write7/1
  OBS TARGETCLASS RECEIVE/1 -> Display35/1, Data Store Write8/1
  OBS THREATCLASS RECEIVE/1 -> Display36/1, Data Store Write9/1
  OBS ID RECEIVE/2 -> Terminator/1
  OBS LATITUDE RECEIVE/2 -> Terminator1/1
  OBS LONGITUDE RECEIVE/2 -> Terminator2/1
  OBS TARGETCLASS RECEIVE/2 -> Terminator3/1
  OBS THREATCLASS RECEIVE/2 -> Terminator4/1
  Constant7/1 -> OBS ID SEND/1
  Constant1/1 -> OBS LATITUDE SEND/1
  Constant2/1 -> OBS LONGITUDE SEND/1
  Constant4/1 -> OBS THREATCLASS SEND/1
  Constant3/1 -> OBS TARGETCLASS SEND/1
  Data Store Read5/1 -> Demux/1
  Demux/1 -> Display7/1
  Demux/2 -> Display8/1
  Demux1/2 -> Display10/1
  Demux1/1 -> Display9/1
  Data Store Read1/1 -> Demux1/1
  Constant5/1 -> Multiport Switch/2
  Constant6/1 -> Multiport Switch1/2
  HUMAN ATT RECEIVE/1 -> Data Store Write3/1, Display11/1
  Data Store Read2/1 -> Display12/1, Scope/1
  HUMAN ATT RECEIVE/2 -> Terminator5/1
  Constant8/1 -> HUMAN ATT SEND/1

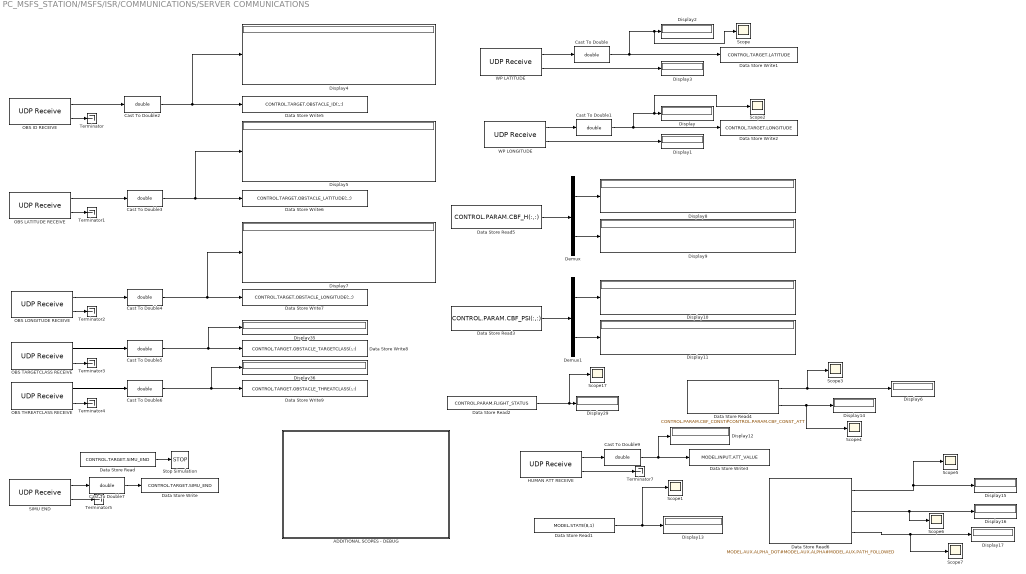
== system PC_MSFS_STATION/MSFS/ISR/COMMUNICATIONS/SERVER COMMUNICATIONS ==
  ADDITIONAL SCOPES - DEBUG : Subsystem
  Cast To Double{,1..7,9} (9 alike) : DataTypeConversion  OutDataTypeStr=double
  Data Store Read : DataStoreRead  DataStoreName=CONTROL  DataStoreElements=CONTROL.TARGET.SIMU_END  IndexOptions=Index vector (dialog)  Indices=1  OutputSizes=1
  Data Store Read1 : DataStoreRead  DataStoreName=MODEL  DataStoreElements=MODEL.STATE(8,1)  IndexOptions=Index vector (dialog)  Indices=1  OutputSizes=1
  Data Store Read2 : DataStoreRead  DataStoreName=CONTROL  DataStoreElements=CONTROL.PARAM.FLIGHT_STATUS  IndexOptions=Index vector (dialog)  Indices=1  OutputSizes=1
  Data Store Read3 : DataStoreRead  DataStoreName=CONTROL  DataStoreElements=CONTROL.PARAM.CBF_PSI(:,:)  IndexOptions=Index vector (dialog)  Indices=1  OutputSizes=1
  Data Store Read4 : DataStoreRead  DataStoreName=CONTROL  DataStoreElements=CONTROL.PARAM.CBF_CONST#CONTROL.PARAM.CBF_CONST_ATT  IndexOptions=Index vector (dialog)  Indices=1  OutputSizes=1
  Data Store Read5 : DataStoreRead  DataStoreName=CONTROL  DataStoreElements=CONTROL.PARAM.CBF_H(:,:)  IndexOptions=Index vector (dialog)  Indices=1  OutputSizes=1
  Data Store Read6 : DataStoreRead  DataStoreName=MODEL  DataStoreElements=MODEL.AUX.ALPHA_DOT#MODEL.AUX.ALPHA#MODEL.AUX.PATH_FOLLOWED  IndexOptions=Index vector (dialog)  Indices=1  OutputSizes=1
  Data Store Write : DataStoreWrite  DataStoreName=CONTROL  DataStoreElements=CONTROL.TARGET.SIMU_END  IndexOptions=Index vector (dialog)  Indices=1  OutputSizes=1
  Data Store Write1 : DataStoreWrite  DataStoreName=CONTROL  DataStoreElements=CONTROL.TARGET.LATITUDE  IndexOptions=Index vector (dialog)  Indices=1  OutputSizes=1
  Data Store Write2 : DataStoreWrite  DataStoreName=CONTROL  DataStoreElements=CONTROL.TARGET.LONGITUDE  IndexOptions=Index vector (dialog)  Indices=1  OutputSizes=1
  Data Store Write3 : DataStoreWrite  DataStoreName=MODEL  DataStoreElements=MODEL.INPUT.ATT_VALUE  IndexOptions=Index vector (dialog)  Indices=1  OutputSizes=1
  Data Store Write5 : DataStoreWrite  DataStoreName=CONTROL  DataStoreElements=CONTROL.TARGET.OBSTACLE_ID(:,:)  IndexOptions=Index vector (dialog)  Indices=1  OutputSizes=1
  Data Store Write6 : DataStoreWrite  DataStoreName=CONTROL  DataStoreElements=CONTROL.TARGET.OBSTACLE_LATITUDE(:,:)  IndexOptions=Index vector (dialog)  Indices=1  OutputSizes=1
  Data Store Write7 : DataStoreWrite  DataStoreName=CONTROL  DataStoreElements=CONTROL.TARGET.OBSTACLE_LONGITUDE(:,:)  IndexOptions=Index vector (dialog)  Indices=1  OutputSizes=1
  Data Store Write8 : DataStoreWrite  DataStoreName=CONTROL  DataStoreElements=CONTROL.TARGET.OBSTACLE_TARGETCLASS(:,:)  IndexOptions=Index vector (dialog)  Indices=1  OutputSizes=1
  Data Store Write9 : DataStoreWrite  DataStoreName=CONTROL  DataStoreElements=CONTROL.TARGET.OBSTACLE_THREATCLASS(:,:)  IndexOptions=Index vector (dialog)  Indices=1  OutputSizes=1
  Demux : Demux  Outputs=2
  Demux1 : Demux  Outputs=2
  Display{,1..17,29,35..36} (21 alike) : Display
  HUMAN ATT RECEIVE : instrumentlib/UDP Receive  Host=127.0.0.1  Port=7083  LocalPort=7082  EnablePortSharing=off  GetLatestData=off  DataSize="[1  1]"  DataType=double  ASCIIFormatting=%f,  Terminator=LF  ByteOrder=BigEndian  EnableBlockingMode=off  Timeout=10  SampleTime=-1  LocalAddress=127.0.0.1
  OBS ID RECEIVE : instrumentlib/UDP Receive  Host=127.0.0.1  Port=8081  LocalPort=8082  EnablePortSharing=off  GetLatestData=off  DataSize="[20   1]"  DataType=double  ASCIIFormatting=%f,  Terminator=LF  ByteOrder=BigEndian  EnableBlockingMode=off  Timeout=10  SampleTime=-1  LocalAddress=127.0.0.1
  OBS LATITUDE RECEIVE : instrumentlib/UDP Receive  Host=127.0.0.1  Port=8083  LocalPort=8084  EnablePortSharing=off  GetLatestData=off  DataSize="[20   1]"  DataType=double  ASCIIFormatting=%f,  Terminator=LF  ByteOrder=BigEndian  EnableBlockingMode=off  Timeout=10  SampleTime=-1  LocalAddress=127.0.0.1
  OBS LONGITUDE RECEIVE : instrumentlib/UDP Receive  Host=127.0.0.1  Port=8085  LocalPort=8086  EnablePortSharing=off  GetLatestData=off  DataSize="[20   1]"  DataType=double  ASCIIFormatting=%f,  Terminator=LF  ByteOrder=BigEndian  EnableBlockingMode=off  Timeout=10  SampleTime=-1  LocalAddress=127.0.0.1
  OBS TARGETCLASS RECEIVE : instrumentlib/UDP Receive  Host=127.0.0.1  Port=7087  LocalPort=7088  EnablePortSharing=off  GetLatestData=off  DataSize="[20   1]"  DataType=double  ASCIIFormatting=%f,  Terminator=LF  ByteOrder=BigEndian  EnableBlockingMode=off  Timeout=10  SampleTime=-1  LocalAddress=127.0.0.1
  OBS THREATCLASS RECEIVE : instrumentlib/UDP Receive  Host=127.0.0.1  Port=7089  LocalPort=7080  EnablePortSharing=off  GetLatestData=off  DataSize="[20   1]"  DataType=double  ASCIIFormatting=%f,  Terminator=LF  ByteOrder=BigEndian  EnableBlockingMode=off  Timeout=10  SampleTime=-1  LocalAddress=127.0.0.1
  SIMU END : instrumentlib/UDP Receive  Host=127.0.0.1  Port=7086  LocalPort=7084  EnablePortSharing=off  GetLatestData=off  DataSize=[1 1]  DataType=single  ASCIIFormatting=%f,  Terminator=LF  ByteOrder=BigEndian  EnableBlockingMode=off  Timeout=10  SampleTime=-1  LocalAddress=127.0.0.1
  Scope{,1..7,17} (9 alike) : Scope
  Stop Simulation : Stop
  Terminator{,1..5,7} (7 alike) : Terminator
  WP LATITUDE : instrumentlib/UDP Receive  Host=127.0.0.1  Port=8081  LocalPort=8080  EnablePortSharing=off  GetLatestData=off  DataSize=[1 1]  DataType=single  ASCIIFormatting=%f,  Terminator=LF  ByteOrder=BigEndian  EnableBlockingMode=off  Timeout=10  SampleTime=-1  LocalAddress=127.0.0.1
  WP LONGITUDE : instrumentlib/UDP Receive  Host=127.0.0.1  Port=8081  LocalPort=8088  EnablePortSharing=off  GetLatestData=off  DataSize=[1 1]  DataType=single  ASCIIFormatting=%f,  Terminator=LF  ByteOrder=BigEndian  EnableBlockingMode=off  Timeout=10  SampleTime=-1  LocalAddress=127.0.0.1
  wires:
  WP LONGITUDE/2 -> Display1/1
  Data Store Read2/1 -> Display29/1, Scope17/1
  WP LATITUDE/2 -> Display3/1
  WP LATITUDE/1 -> Cast To Double/1
  Cast To Double/1 -> Scope/1, Display2/1, Data Store Write1/1
  WP LONGITUDE/1 -> Cast To Double1/1
  Cast To Double1/1 -> Scope2/1, Display/1, Data Store Write2/1
  OBS LATITUDE RECEIVE/1 -> Cast To Double3/1
  OBS THREATCLASS RECEIVE/1 -> Cast To Double6/1
  OBS TARGETCLASS RECEIVE/2 -> Terminator3/1
  OBS LONGITUDE RECEIVE/2 -> Terminator2/1
  OBS LATITUDE RECEIVE/2 -> Terminator1/1
  OBS ID RECEIVE/2 -> Terminator/1
  OBS LONGITUDE RECEIVE/1 -> Cast To Double4/1
  OBS TARGETCLASS RECEIVE/1 -> Cast To Double5/1
  OBS THREATCLASS RECEIVE/2 -> Terminator4/1
  Cast To Double3/1 -> Display5/1, Data Store Write6/1
  Cast To Double4/1 -> Display7/1, Data Store Write7/1
  Cast To Double5/1 -> Display35/1, Data Store Write8/1
  Cast To Double6/1 -> Display36/1, Data Store Write9/1
  Data Store Read/1 -> Stop Simulation/1
  SIMU END/2 -> Terminator5/1
  SIMU END/1 -> Cast To Double7/1
  Cast To Double7/1 -> Data Store Write/1
  OBS ID RECEIVE/1 -> Cast To Double2/1
  Cast To Double2/1 -> Data Store Write5/1, Display4/1
  Demux/1 -> Display8/1
  Demux/2 -> Display9/1
  Data Store Read5/1 -> Demux/1
  Data Store Read3/1 -> Demux1/1
  Demux1/2 -> Display11/1
  Demux1/1 -> Display10/1
  Cast To Double9/1 -> Display12/1, Data Store Write3/1
  HUMAN ATT RECEIVE/1 -> Cast To Double9/1
  HUMAN ATT RECEIVE/2 -> Terminator7/1
  Data Store Read1/1 -> Display13/1, Scope1/1
  Data Store Read4/1 -> Display6/1, Scope3/1
  Data Store Read4/2 -> Scope4/1, Display14/1
  Data Store Read6/1 -> Scope5/1, Display15/1
  Data Store Read6/2 -> Display16/1, Scope6/1
  Data Store Read6/3 -> Display17/1, Scope7/1
